simulink model "double_lwa4p_platform"  (R2020b)
settings: Solver=ode15s  StartTime=0.0  StopTime=T  MaxStep=0.01  RelTol=1e-3
values from neighbouring files (symbols this model uses):
  F_ee = [F_ee_A F_ee_B]    [sim_double_lwa4p_platform.m]
  friction = [fv1 fv2 fv3 fv4 fv5 fv6 fv1 fv2 fv3 fv4 fv5 fv6]    [sim_double_lwa4p_platform.m]
  g = [0 0 g0]'    [sim_double_lwa4p_platform.m]
  Kd = 5*eye(12)    [sim_double_lwa4p_platform.m]
  Kp = 2*eye(12)    [sim_double_lwa4p_platform.m]
  mass = [ml1 ml2 ml3 ml4 ml5 ml6 ml1 ml2 ml3 ml4 ml5 ml6]    [sim_double_lwa4p_platform.m]
  n_joints = 6    [sim_double_lwa4p_platform.m]
  q_ref = [pi/2 pi/4 pi/2 -pi/2 pi/2 -pi/8 pi/2 pi/4 pi/2 -pi/2 pi/2 -pi/8]    [sim_double_lwa4p_platform.m]
  qd_ref = zeros(1,12)    [sim_double_lwa4p_platform.m]
  qdd_ref = zeros(1,12)    [sim_double_lwa4p_platform.m]
  S = [S_A S_B]    [sim_double_lwa4p_platform.m]
  th1A_0 = deg2rad(0)    [sim_double_lwa4p_platform.m]
  th1B_0 = deg2rad(0)    [sim_double_lwa4p_platform.m]
  th2A_0 = deg2rad(0)    [sim_double_lwa4p_platform.m]
  th2B_0 = deg2rad(0)    [sim_double_lwa4p_platform.m]
  th3A_0 = deg2rad(0)    [sim_double_lwa4p_platform.m]
  th3B_0 = deg2rad(0)    [sim_double_lwa4p_platform.m]
  th4A_0 = deg2rad(0)    [sim_double_lwa4p_platform.m]
  th4B_0 = deg2rad(0)    [sim_double_lwa4p_platform.m]
  th5A_0 = deg2rad(0)    [sim_double_lwa4p_platform.m]
  th5B_0 = deg2rad(0)    [sim_double_lwa4p_platform.m]
  th6A_0 = deg2rad(0)    [sim_double_lwa4p_platform.m]
  th6B_0 = deg2rad(0)    [sim_double_lwa4p_platform.m]
undefined symbols (not defined in the file or in its folder): g0, Inertia, inertial_disp, ixx_1, ixx_2, ixx_3, ixx_4, ixx_5, ixx_6, ixx_platform, ixy_1, ixy_2, ixy_3, ixy_4, ixy_5, ixy_6, ixy_platform, ixz_1, ixz_2, ixz_3, ixz_4, ixz_5, ixz_6, ixz_platform, iyy_1, iyy_2, iyy_3, iyy_4, iyy_5, iyy_6, iyy_platform, iyz_1, iyz_2, iyz_3, iyz_4, iyz_5, iyz_6, iyz_platform, izz_1, izz_2, izz_3, izz_4, izz_5, izz_6, izz_platform, M_bi, m_platform, ml1, ml2, ml3, ml4, ml5, ml6, offA, offB, X, Y, Z
libraries: sm_lib x118, nesl_utility x49
(part 1 of 3)
settings Model: Creator=giank  LastModifiedBy=giank
settings ExplorerConfigSet: InternalSimMechanicsExplorerSettings="<ExplorerConfiguration><canonicalview>default</canonicalview><AnimationSetting><BasePlaybackSpeed>1.0</BasePlaybackSpeed><PlaybackSpeedFactor>1.0</PlaybackSpeedFactor></AnimationSetting><TilePanel><TileInfo><Tiles Columns=\"2\" Count=\"2\" Rows=\"1\"><Column Weight=\"0.4996\"/><Column Weight=\"0.5004\"/><Row Weight=\"1\"/><Tile Height=\"1\" Width=\"1\" X=\"0\" Y=\"0\"/><Tile Height=\"1\" Width=\"1\" X=\"1\" Y=\"0\"/></Tiles></TileInfo><SceneInfo><SceneViewer><BGColor><R>0.60000002384185791</R><G>0.60000002384185791</G><B>0.60000002384185791</B></BGColor><Camera><DoPerspective>off</DoPerspective><Position><X>-1.1818962679743017</X><Y>0.00783108174800895007</Y><Z>-0.680611997842788474</Z></Position><Center><X>1.20246335295615125e-05</X><Y>0.00783108174800895007</Y><Z>-0.680611997842788474</Z></Center><Up><X>0</X><Y>0</Y><Z>1</Z></Up><ViewLimDist>1</ViewLimDist><YLim>1.07089078664779658</YLim><XLim>0.814025905030074881</XLim></Camera></SceneViewer><SceneViewer><BGColor><R>0.60000002384185791</R><G>0.60000002384185791</G><B>0.60000002384185791</B></BGColor><Camera><DoPerspective>off</DoPerspective><Position><X>1.20351777254112946e-05</X><Y>-1.17407721146337618</Y><Z>-0.680611991448779152</Z></Position><Center><X>1.20351777254112946e-05</X><Y>0.00783108114445518755</Y><Z>-0.680611991448779152</Z></Center><Up><X>0</X><Y>-0</Y><Z>1</Z></Up><ViewLimDist>1</ViewLimDist><YLim>1.07089078664779658</YLim><XLim>0.816507691325898177</XLim></Camera></SceneViewer></SceneInfo></TilePanel><MechEditorPanel><Cameras/><GfxPanelCameraMap/><VideoCreator><PlaybackSpeedRatio>1.0</PlaybackSpeedRatio><FrameRate>30</FrameRate><VideoFormat>Motion JPEG AVI</VideoFormat><FrameSize>auto</FrameSize></VideoCreator></MechEditorPanel></ExplorerConfiguration>"

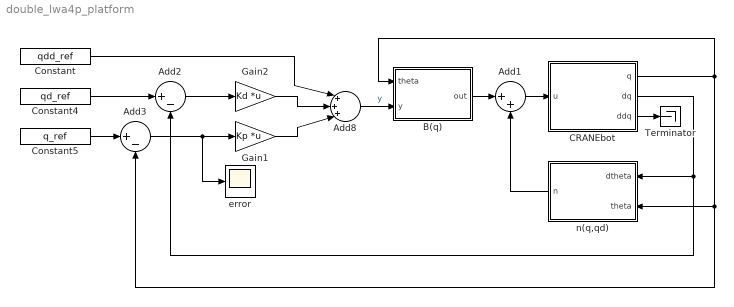
== system double_lwa4p_platform ==
  Add1 : Sum  Inputs=|++
  Add2 : Sum  Inputs=|+-
  Add3 : Sum  Inputs=|+-
  Add8 : Sum  Inputs=|+++|
  B(q) : MATLAB Function  TreatAsAtomicUnit=on
  CRANEbot : Subsystem
  Constant : Constant  Value=qdd_ref
  Constant4 : Constant  Value=qd_ref
  Constant5 : Constant  Value=q_ref
  Gain1 : Gain  Gain=Kp  Multiplication=Matrix(K*u)
  Gain2 : Gain  Gain=Kd  Multiplication=Matrix(K*u)
  Terminator : Terminator
  error : Scope
  n(q,qd) : MATLAB Function  TreatAsAtomicUnit=on
  wires:
  Gain1/1 -> Add8/3
  Add1/1 -> CRANEbot/1(u)
  CRANEbot/3(ddq) -> Terminator/1
  CRANEbot/2(dq) -> n(q,qd)/1(dtheta), Add2/2
  n(q,qd)/1(n) -> Add1/2
  Constant5/1 -> Add3/1
  B(q)/1(out) -> Add1/1
  Add8/1 -> B(q)/2(y)  "y"
  Constant4/1 -> Add2/1
  CRANEbot/1(q) -> n(q,qd)/2(theta), Add3/2, B(q)/1(theta)
  Add3/1 -> Gain1/1, error/1
  Constant/1 -> Add8/1
  Add2/1 -> Gain2/1
  Gain2/1 -> Add8/2

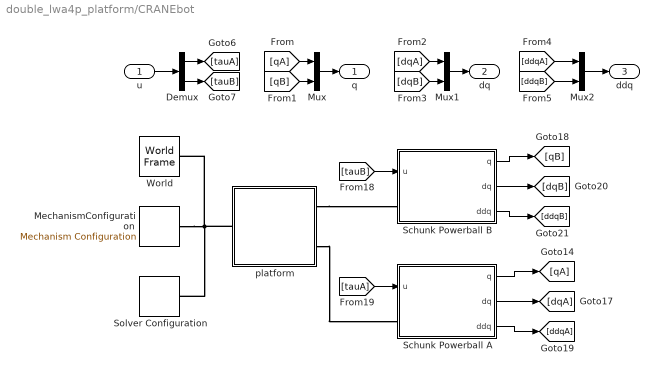
== system double_lwa4p_platform/CRANEbot ==
  u : Inport
  Demux : Demux  Outputs=[6 6 ]
  MechanismConfiguration : sm_lib/Utilities/Mechanism Configuration  UniformGravity=Constant  GravityVector=[0 0 -g0]  GravityVectorUnits=m/s^2  GravityUnits=m/s^2  LinearizationDelta=0.001  JointModeTransitionNonlinearIterations=2
  Mux : Mux  Inputs=[6 6]
  Mux1 : Mux  Inputs=[6 6]
  Mux2 : Mux  Inputs=[6 6]
  Schunk Powerball A : Subsystem  mask{th1_0=th1A_0, th2_0=th2A_0, th3_0=th3A_0, th4_0=th4A_0, th5_0=th5A_0, th6_0=th6A_0}
      mask prompts: th1_0 "th1_0 (rad)"; th2_0 "th2_0 (rad)"; th3_0 "th3_0 (rad)"; th4_0 "th4_0 (rad)"; th5_0 "th5_0 (rad)"; th6_0 "th6_0 (rad)"
  Schunk Powerball B : Subsystem  mask{th1_0=th1B_0, th2_0=th2B_0, th3_0=th3B_0, th4_0=th4B_0, th5_0=th5B_0, th6_0=th6B_0}
      mask prompts: th1_0 "th1_0 (rad)"; th2_0 "th2_0 (rad)"; th3_0 "th3_0 (rad)"; th4_0 "th4_0 (rad)"; th5_0 "th5_0 (rad)"; th6_0 "th6_0 (rad)"
  Solver Configuration : nesl_utility/Solver Configuration  PhysicalDomain=network_engine_domain  SubClassName=solver  LeftPortType=input  RightPortType=generic  Tones=[]  Harmonics=[]  SimulateNoise=off  Profile=off  UseLocalSampling=off  EnableSwitchedLinearOptims=on  FrequencyDomain=off  UseCCode=off  RelTol=0.001  AbsTol=1e-06  MinStep=1e-09  ToWorkspace=off  RevertToSquareIcSolve=off  NumHomotopyIterations=100  PhasorMode=off  PhasorModeNumHarmonics=1  DoDC=off  ResidualTolerance=1e-09  UseLocalSolver=off  LocalSolverChoice=NE_BACKWARD_EULER_ADVANCER  LocalSolverSampleTime=0.001  DoFixedCost=off  MaxNonlinIter=3  MaxModeIter=2  ComputeImpulses=off  ImpulseIterations=2  LinearAlgebra=auto  EquationFormulation=NE_TIME_EF  DelaysMemoryBudget=1024  AutomaticFiltering=on  FilteringTimeConstant=0.001  PartitionStorageMethod=AS_NEEDED  PartitionMemoryBudget=1024  PartitionMethod=ROBUST
  World : sm_lib/Frames and Transforms/World Frame
  platform : Subsystem
  q : Outport
  dq : Outport  Port=2
  ddq : Outport  Port=3
  wires:
  Mux/1 -> q/1
  [qA] -> Mux/1
  Mux1/1 -> dq/1
  u/1 -> Demux/1
  [qB] -> Mux/2
  Demux/1 -> [tauA]
  [dqB] -> Mux1/2
  Demux/2 -> [tauB]
  Mux2/1 -> ddq/1
  [ddqA] -> Mux2/1
  [dqA] -> Mux1/1
  [ddqB] -> Mux2/2
  Schunk Powerball B/2(dq) -> [dqB]
  Schunk Powerball A/1(q) -> [qA]
  Schunk Powerball B/3(ddq) -> [ddqB]
  Schunk Powerball A/2(dq) -> [dqA]
  [tauB] -> Schunk Powerball B/1(u)
  Schunk Powerball A/3(ddq) -> [ddqA]
  [tauA] -> Schunk Powerball A/1(u)
  Schunk Powerball B/1(q) -> [qB]
  connections:
  Solver Configuration/RConn1 -- platform/LConn1 -- World/RConn1 -- MechanismConfiguration/RConn1
  platform/RConn1 -- Schunk Powerball B/LConn1
  platform/RConn2 -- Schunk Powerball A/LConn1

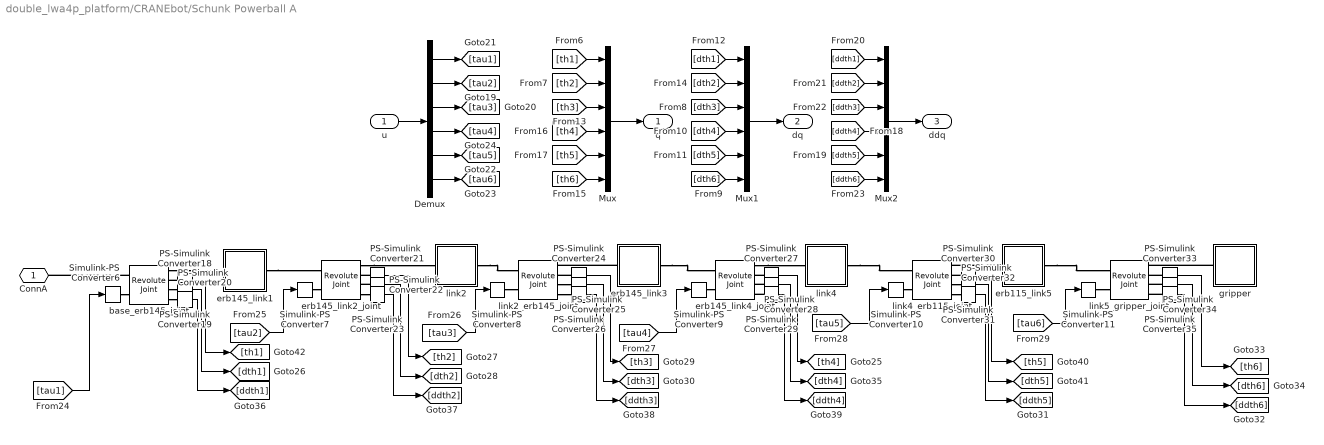
== system double_lwa4p_platform/CRANEbot/Schunk Powerball A ==
  u : Inport
  Demux : Demux  Outputs=6
  Mux : Mux  Inputs=6
  Mux1 : Mux  Inputs=6
  Mux2 : Mux  Inputs=6
  PS-Simulink Converter{18..35} (18 alike) : nesl_utility/PS-Simulink Converter  PhysicalDomain=network_engine_domain  SubClassName=ps_output  LeftPortType=input  RightPortType=output  PseudoPeriodic=off  Frequencies=[]  Unit=inherit  AffineConversion=off
  Simulink-PS Converter{6..11} (6 alike) : nesl_utility/Simulink-PS Converter  PhysicalDomain=network_engine_domain  SubClassName=ps_input  LeftPortType=input  RightPortType=output  PseudoPeriodic=off  Frequencies=[]  NoiseDistribution=none  NoiseParameters=[]  Unit=1  AffineConversion=off  FilteringAndDerivatives=provide  SimscapeFilterOrder=1  InputFilterTimeConstant=0.001  UdotUserProvided=0
  base_erb145_joint : sm_lib/Joints/Revolute Joint  JointMode=Normal  SenseConstraintForce=off  SenseConstraintForceX=off  SenseConstraintForceY=off  SenseConstraintForceZ=off  SenseConstraintTorque=off  SenseConstraintTorqueX=off  SenseConstraintTorqueY=off  SenseConstraintTorqueZ=off  SenseTotalForce=off  SenseTotalForceX=off  SenseTotalForceY=off  SenseTotalForceZ=off  SenseTotalTorque=off  SenseTotalTorqueX=off  SenseTotalTorqueY=off  SenseTotalTorqueZ=off  CompositeWrenchDir=FollowerOnBase  CompositeWrenchFrame=BaseFrame  EquilibriumPosition=0  EquilibriumPositionUnits=deg  SpringStiffness=0  SpringStiffnessUnits=N*m/deg  DampingCoefficient=fv1  DampingCoefficientUnits=N*m/(rad/s)  TorqueActuationMode=InputTorque  MotionActuationMode=ComputedMotion  SensePosition=on  SenseVelocity=on  SenseAcceleration=on  SenseTorqueForce=off  SenseLowerLimitTorqueForce=off  SenseUpperLimitTorqueForce=off  LowerLimitSpecify=on  LowerLimitBound=J1_lower_limit  LowerLimitBoundUnits=deg  LowerLimitStiffness=1e4  LowerLimitStiffnessUnits=N*m/deg  LowerLimitDamping=10  LowerLimitDampingUnits=N*m/(deg/s)  LowerLimitTransitionRegionWidth=0.1  LowerLimitTransitionRegionWidthUnits=deg  UpperLimitSpecify=on  UpperLimitBound=J1_upper_limit  UpperLimitBoundUnits=deg  UpperLimitStiffness=1e4  UpperLimitStiffnessUnits=N*m/deg  UpperLimitDamping=10  UpperLimitDampingUnits=N*m/(deg/s)  UpperLimitTransitionRegionWidth=0.1  UpperLimitTransitionRegionWidthUnits=deg  PositionTargetSpecify=on  PositionTargetPriority=High  PositionTargetValue=th1_0  PositionTargetValueUnits=rad  VelocityTargetSpecify=off  VelocityTargetPriority=High  VelocityTargetValue=0  VelocityTargetValueUnits=deg/s
  erb115_link5 : Subsystem
  erb145_link1 : Subsystem
  erb145_link2_joint : sm_lib/Joints/Revolute Joint  JointMode=Normal  SenseConstraintForce=off  SenseConstraintForceX=off  SenseConstraintForceY=off  SenseConstraintForceZ=off  SenseConstraintTorque=off  SenseConstraintTorqueX=off  SenseConstraintTorqueY=off  SenseConstraintTorqueZ=off  SenseTotalForce=off  SenseTotalForceX=off  SenseTotalForceY=off  SenseTotalForceZ=off  SenseTotalTorque=off  SenseTotalTorqueX=off  SenseTotalTorqueY=off  SenseTotalTorqueZ=off  CompositeWrenchDir=FollowerOnBase  CompositeWrenchFrame=BaseFrame  EquilibriumPosition=0  EquilibriumPositionUnits=deg  SpringStiffness=0  SpringStiffnessUnits=N*m/deg  DampingCoefficient=fv2  DampingCoefficientUnits=N*m/(rad/s)  TorqueActuationMode=InputTorque  MotionActuationMode=ComputedMotion  SensePosition=on  SenseVelocity=on  SenseAcceleration=on  SenseTorqueForce=off  SenseLowerLimitTorqueForce=off  SenseUpperLimitTorqueForce=off  LowerLimitSpecify=on  LowerLimitBound=J2_lower_limit  LowerLimitBoundUnits=deg  LowerLimitStiffness=1e4  LowerLimitStiffnessUnits=N*m/deg  LowerLimitDamping=10  LowerLimitDampingUnits=N*m/(deg/s)  LowerLimitTransitionRegionWidth=0.1  LowerLimitTransitionRegionWidthUnits=deg  UpperLimitSpecify=on  UpperLimitBound=J2_upper_limit  UpperLimitBoundUnits=deg  UpperLimitStiffness=1e4  UpperLimitStiffnessUnits=N*m/deg  UpperLimitDamping=10  UpperLimitDampingUnits=N*m/(deg/s)  UpperLimitTransitionRegionWidth=0.1  UpperLimitTransitionRegionWidthUnits=deg  PositionTargetSpecify=on  PositionTargetPriority=High  PositionTargetValue=th2_0  PositionTargetValueUnits=deg  VelocityTargetSpecify=off  VelocityTargetPriority=High  VelocityTargetValue=0  VelocityTargetValueUnits=deg/s
  erb145_link3 : Subsystem
  erb145_link4_joint : sm_lib/Joints/Revolute Joint  JointMode=Normal  SenseConstraintForce=off  SenseConstraintForceX=off  SenseConstraintForceY=off  SenseConstraintForceZ=off  SenseConstraintTorque=off  SenseConstraintTorqueX=off  SenseConstraintTorqueY=off  SenseConstraintTorqueZ=off  SenseTotalForce=off  SenseTotalForceX=off  SenseTotalForceY=off  SenseTotalForceZ=off  SenseTotalTorque=off  SenseTotalTorqueX=off  SenseTotalTorqueY=off  SenseTotalTorqueZ=off  CompositeWrenchDir=FollowerOnBase  CompositeWrenchFrame=BaseFrame  EquilibriumPosition=0  EquilibriumPositionUnits=deg  SpringStiffness=0  SpringStiffnessUnits=N*m/deg  DampingCoefficient=fv4  DampingCoefficientUnits=N*m/(rad/s)  TorqueActuationMode=InputTorque  MotionActuationMode=ComputedMotion  SensePosition=on  SenseVelocity=on  SenseAcceleration=on  SenseTorqueForce=off  SenseLowerLimitTorqueForce=off  SenseUpperLimitTorqueForce=off  LowerLimitSpecify=on  LowerLimitBound=J4_lower_limit  LowerLimitBoundUnits=deg  LowerLimitStiffness=1e4  LowerLimitStiffnessUnits=N*m/deg  LowerLimitDamping=10  LowerLimitDampingUnits=N*m/(deg/s)  LowerLimitTransitionRegionWidth=0.1  LowerLimitTransitionRegionWidthUnits=deg  UpperLimitSpecify=on  UpperLimitBound=J4_upper_limit  UpperLimitBoundUnits=deg  UpperLimitStiffness=1e4  UpperLimitStiffnessUnits=N*m/deg  UpperLimitDamping=10  UpperLimitDampingUnits=N*m/(deg/s)  UpperLimitTransitionRegionWidth=0.1  UpperLimitTransitionRegionWidthUnits=deg  PositionTargetSpecify=on  PositionTargetPriority=High  PositionTargetValue=th4_0  PositionTargetValueUnits=deg  VelocityTargetSpecify=off  VelocityTargetPriority=High  VelocityTargetValue=0  VelocityTargetValueUnits=deg/s
  gripper : Subsystem
  link2 : Subsystem
  link2_erb145_joint : sm_lib/Joints/Revolute Joint  JointMode=Normal  SenseConstraintForce=off  SenseConstraintForceX=off  SenseConstraintForceY=off  SenseConstraintForceZ=off  SenseConstraintTorque=off  SenseConstraintTorqueX=off  SenseConstraintTorqueY=off  SenseConstraintTorqueZ=off  SenseTotalForce=off  SenseTotalForceX=off  SenseTotalForceY=off  SenseTotalForceZ=off  SenseTotalTorque=off  SenseTotalTorqueX=off  SenseTotalTorqueY=off  SenseTotalTorqueZ=off  CompositeWrenchDir=FollowerOnBase  CompositeWrenchFrame=BaseFrame  EquilibriumPosition=0  EquilibriumPositionUnits=deg  SpringStiffness=0  SpringStiffnessUnits=N*m/deg  DampingCoefficient=fv3  DampingCoefficientUnits=N*m/(rad/s)  TorqueActuationMode=InputTorque  MotionActuationMode=ComputedMotion  SensePosition=on  SenseVelocity=on  SenseAcceleration=on  SenseTorqueForce=off  SenseLowerLimitTorqueForce=off  SenseUpperLimitTorqueForce=off  LowerLimitSpecify=on  LowerLimitBound=J3_lower_limit  LowerLimitBoundUnits=deg  LowerLimitStiffness=1e4  LowerLimitStiffnessUnits=N*m/deg  LowerLimitDamping=10  LowerLimitDampingUnits=N*m/(deg/s)  LowerLimitTransitionRegionWidth=0.1  LowerLimitTransitionRegionWidthUnits=deg  UpperLimitSpecify=on  UpperLimitBound=J3_upper_limit  UpperLimitBoundUnits=deg  UpperLimitStiffness=1e4  UpperLimitStiffnessUnits=N*m/deg  UpperLimitDamping=10  UpperLimitDampingUnits=N*m/(deg/s)  UpperLimitTransitionRegionWidth=0.1  UpperLimitTransitionRegionWidthUnits=deg  PositionTargetSpecify=on  PositionTargetPriority=High  PositionTargetValue=th3_0  PositionTargetValueUnits=deg  VelocityTargetSpecify=off  VelocityTargetPriority=High  VelocityTargetValue=0  VelocityTargetValueUnits=deg/s
  link4 : Subsystem
  link4_erb115_joint : sm_lib/Joints/Revolute Joint  JointMode=Normal  SenseConstraintForce=off  SenseConstraintForceX=off  SenseConstraintForceY=off  SenseConstraintForceZ=off  SenseConstraintTorque=off  SenseConstraintTorqueX=off  SenseConstraintTorqueY=off  SenseConstraintTorqueZ=off  SenseTotalForce=off  SenseTotalForceX=off  SenseTotalForceY=off  SenseTotalForceZ=off  SenseTotalTorque=off  SenseTotalTorqueX=off  SenseTotalTorqueY=off  SenseTotalTorqueZ=off  CompositeWrenchDir=FollowerOnBase  CompositeWrenchFrame=BaseFrame  EquilibriumPosition=0  EquilibriumPositionUnits=deg  SpringStiffness=0  SpringStiffnessUnits=N*m/deg  DampingCoefficient=fv5  DampingCoefficientUnits=N*m/(rad/s)  TorqueActuationMode=InputTorque  MotionActuationMode=ComputedMotion  SensePosition=on  SenseVelocity=on  SenseAcceleration=on  SenseTorqueForce=off  SenseLowerLimitTorqueForce=off  SenseUpperLimitTorqueForce=off  LowerLimitSpecify=on  LowerLimitBound=J5_lower_limit  LowerLimitBoundUnits=deg  LowerLimitStiffness=1e4  LowerLimitStiffnessUnits=N*m/deg  LowerLimitDamping=10  LowerLimitDampingUnits=N*m/(deg/s)  LowerLimitTransitionRegionWidth=0.1  LowerLimitTransitionRegionWidthUnits=deg  UpperLimitSpecify=on  UpperLimitBound=J5_upper_limit  UpperLimitBoundUnits=deg  UpperLimitStiffness=1e4  UpperLimitStiffnessUnits=N*m/deg  UpperLimitDamping=10  UpperLimitDampingUnits=N*m/(deg/s)  UpperLimitTransitionRegionWidth=0.1  UpperLimitTransitionRegionWidthUnits=deg  PositionTargetSpecify=on  PositionTargetPriority=High  PositionTargetValue=th5_0  PositionTargetValueUnits=deg  VelocityTargetSpecify=off  VelocityTargetPriority=High  VelocityTargetValue=0  VelocityTargetValueUnits=deg/s
  link5_gripper_joint : sm_lib/Joints/Revolute Joint  JointMode=Normal  SenseConstraintForce=off  SenseConstraintForceX=off  SenseConstraintForceY=off  SenseConstraintForceZ=off  SenseConstraintTorque=off  SenseConstraintTorqueX=off  SenseConstraintTorqueY=off  SenseConstraintTorqueZ=off  SenseTotalForce=off  SenseTotalForceX=off  SenseTotalForceY=off  SenseTotalForceZ=off  SenseTotalTorque=off  SenseTotalTorqueX=off  SenseTotalTorqueY=off  SenseTotalTorqueZ=off  CompositeWrenchDir=FollowerOnBase  CompositeWrenchFrame=BaseFrame  EquilibriumPosition=0  EquilibriumPositionUnits=deg  SpringStiffness=0  SpringStiffnessUnits=N*m/deg  DampingCoefficient=fv6  DampingCoefficientUnits=N*m/(rad/s)  TorqueActuationMode=InputTorque  MotionActuationMode=ComputedMotion  SensePosition=on  SenseVelocity=on  SenseAcceleration=on  SenseTorqueForce=off  SenseLowerLimitTorqueForce=off  SenseUpperLimitTorqueForce=off  LowerLimitSpecify=on  LowerLimitBound=J6_lower_limit  LowerLimitBoundUnits=deg  LowerLimitStiffness=1e4  LowerLimitStiffnessUnits=N*m/deg  LowerLimitDamping=10  LowerLimitDampingUnits=N*m/(deg/s)  LowerLimitTransitionRegionWidth=0.1  LowerLimitTransitionRegionWidthUnits=deg  UpperLimitSpecify=on  UpperLimitBound=J6_upper_limit  UpperLimitBoundUnits=deg  UpperLimitStiffness=1e4  UpperLimitStiffnessUnits=N*m/deg  UpperLimitDamping=10  UpperLimitDampingUnits=N*m/(deg/s)  UpperLimitTransitionRegionWidth=0.1  UpperLimitTransitionRegionWidthUnits=deg  PositionTargetSpecify=on  PositionTargetPriority=High  PositionTargetValue=th6_0  PositionTargetValueUnits=deg  VelocityTargetSpecify=off  VelocityTargetPriority=High  VelocityTargetValue=0  VelocityTargetValueUnits=deg/s
  ConnA : PMIOPort  Side=Left
  q : Outport
  dq : Outport  Port=2
  ddq : Outport  Port=3
  wires:
  [tau6] -> Simulink-PS Converter11/1
  PS-Simulink Converter22/1 -> [dth2]
  Demux/2 -> [tau2]
  [ddth6] -> Mux2/6
  PS-Simulink Converter28/1 -> [dth4]
  [dth2] -> Mux1/2
  Demux/5 -> [tau5]
  [tau4] -> Simulink-PS Converter9/1
  PS-Simulink Converter30/1 -> [th5]
  PS-Simulink Converter19/1 -> [dth1]
  [th3] -> Mux/3
  PS-Simulink Converter34/1 -> [dth6]
  PS-Simulink Converter26/1 -> [ddth3]
  PS-Simulink Converter24/1 -> [th3]
  PS-Simulink Converter25/1 -> [dth3]
  PS-Simulink Converter31/1 -> [dth5]
  PS-Simulink Converter27/1 -> [th4]
  [dth3] -> Mux1/3
  [th1] -> Mux/1
  PS-Simulink Converter33/1 -> [th6]
  u/1 -> Demux/1
  [th2] -> Mux/2
  [ddth3] -> Mux2/3
  Demux/6 -> [tau6]
  PS-Simulink Converter20/1 -> [ddth1]
  Mux/1 -> q/1
  PS-Simulink Converter18/1 -> [th1]
  [ddth4] -> Mux2/4
  PS-Simulink Converter29/1 -> [ddth4]
  [ddth2] -> Mux2/2
  [dth1] -> Mux1/1
  [dth5] -> Mux1/5
  Demux/4 -> [tau4]
  [dth4] -> Mux1/4
  [dth6] -> Mux1/6
  PS-Simulink Converter23/1 -> [ddth2]
  [th5] -> Mux/5
  [ddth5] -> Mux2/5
  [th4] -> Mux/4
  Mux2/1 -> ddq/1
  PS-Simulink Converter21/1 -> [th2]
  Mux1/1 -> dq/1
  [ddth1] -> Mux2/1
  Demux/3 -> [tau3]
  PS-Simulink Converter32/1 -> [ddth5]
  [tau2] -> Simulink-PS Converter7/1
  [tau3] -> Simulink-PS Converter8/1
  Demux/1 -> [tau1]
  [tau5] -> Simulink-PS Converter10/1
  [tau1] -> Simulink-PS Converter6/1
  PS-Simulink Converter35/1 -> [ddth6]
  [th6] -> Mux/6
  connections:
  erb145_link1/RConn1 -- erb145_link2_joint/LConn1
  erb115_link5/RConn1 -- link5_gripper_joint/LConn1
  Simulink-PS Converter9/RConn1 -- erb145_link4_joint/LConn2
  base_erb145_joint/LConn1 -- ConnA/RConn1
  base_erb145_joint/RConn1 -- erb145_link1/LConn1
  Simulink-PS Converter7/RConn1 -- erb145_link2_joint/LConn2
  PS-Simulink Converter18/LConn1 -- base_erb145_joint/RConn2
  erb145_link3/LConn1 -- link2_erb145_joint/RConn1
  Simulink-PS Converter6/RConn1 -- base_erb145_joint/LConn2
  link2_erb145_joint/RConn3 -- PS-Simulink Converter25/LConn1
  link2_erb145_joint/RConn4 -- PS-Simulink Converter26/LConn1
  PS-Simulink Converter21/LConn1 -- erb145_link2_joint/RConn2
  PS-Simulink Converter33/LConn1 -- link5_gripper_joint/RConn2
  PS-Simulink Converter22/LConn1 -- erb145_link2_joint/RConn3
  link2/RConn1 -- link2_erb145_joint/LConn1
  Simulink-PS Converter8/RConn1 -- link2_erb145_joint/LConn2
  erb115_link5/LConn1 -- link4_erb115_joint/RConn1
  erb145_link2_joint/RConn1 -- link2/LConn1
  PS-Simulink Converter28/LConn1 -- erb145_link4_joint/RConn3
  PS-Simulink Converter35/LConn1 -- link5_gripper_joint/RConn4
  PS-Simulink Converter29/LConn1 -- erb145_link4_joint/RConn4
  Simulink-PS Converter10/RConn1 -- link4_erb115_joint/LConn2
  PS-Simulink Converter30/LConn1 -- link4_erb115_joint/RConn2
  base_erb145_joint/RConn3 -- PS-Simulink Converter19/LConn1
  erb145_link2_joint/RConn4 -- PS-Simulink Converter23/LConn1
  link4/RConn1 -- link4_erb115_joint/LConn1
  link4_erb115_joint/RConn4 -- PS-Simulink Converter32/LConn1
  erb145_link4_joint/RConn1 -- link4/LConn1
  PS-Simulink Converter24/LConn1 -- link2_erb145_joint/RConn2
  Simulink-PS Converter11/RConn1 -- link5_gripper_joint/LConn2
  PS-Simulink Converter34/LConn1 -- link5_gripper_joint/RConn3
  erb145_link3/RConn1 -- erb145_link4_joint/LConn1
  PS-Simulink Converter27/LConn1 -- erb145_link4_joint/RConn2
  link4_erb115_joint/RConn3 -- PS-Simulink Converter31/LConn1
  gripper/LConn1 -- link5_gripper_joint/RConn1
  base_erb145_joint/RConn4 -- PS-Simulink Converter20/LConn1

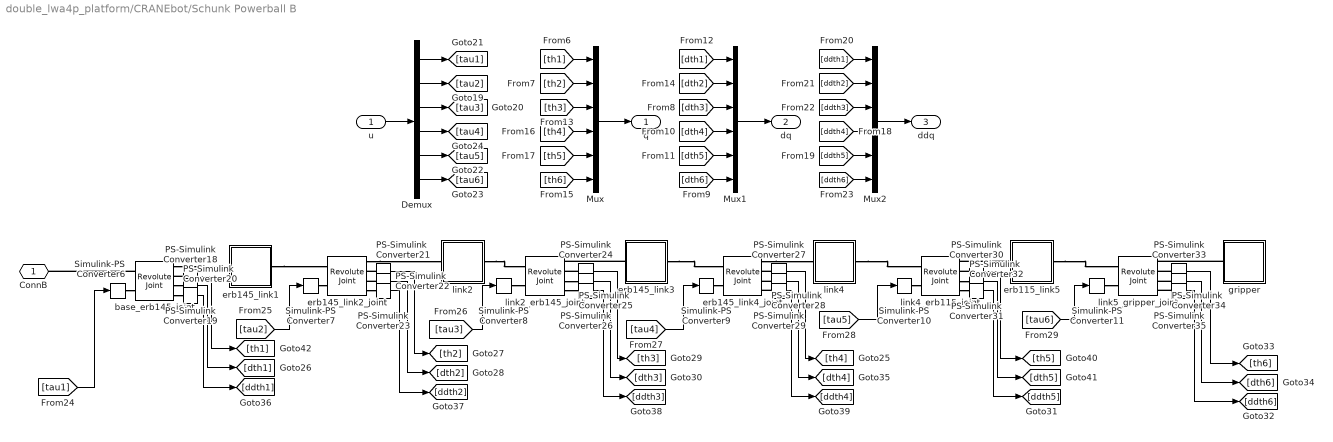
== system double_lwa4p_platform/CRANEbot/Schunk Powerball B ==
  u : Inport
  Demux : Demux  Outputs=6
  Mux : Mux  Inputs=6
  Mux1 : Mux  Inputs=6
  Mux2 : Mux  Inputs=6
  PS-Simulink Converter{18..35} (18 alike) : nesl_utility/PS-Simulink Converter  PhysicalDomain=network_engine_domain  SubClassName=ps_output  LeftPortType=input  RightPortType=output  PseudoPeriodic=off  Frequencies=[]  Unit=inherit  AffineConversion=off
  Simulink-PS Converter{6..11} (6 alike) : nesl_utility/Simulink-PS Converter  PhysicalDomain=network_engine_domain  SubClassName=ps_input  LeftPortType=input  RightPortType=output  PseudoPeriodic=off  Frequencies=[]  NoiseDistribution=none  NoiseParameters=[]  Unit=1  AffineConversion=off  FilteringAndDerivatives=provide  SimscapeFilterOrder=1  InputFilterTimeConstant=0.001  UdotUserProvided=0
  base_erb145_joint : sm_lib/Joints/Revolute Joint  JointMode=Normal  SenseConstraintForce=off  SenseConstraintForceX=off  SenseConstraintForceY=off  SenseConstraintForceZ=off  SenseConstraintTorque=off  SenseConstraintTorqueX=off  SenseConstraintTorqueY=off  SenseConstraintTorqueZ=off  SenseTotalForce=off  SenseTotalForceX=off  SenseTotalForceY=off  SenseTotalForceZ=off  SenseTotalTorque=off  SenseTotalTorqueX=off  SenseTotalTorqueY=off  SenseTotalTorqueZ=off  CompositeWrenchDir=FollowerOnBase  CompositeWrenchFrame=BaseFrame  EquilibriumPosition=0  EquilibriumPositionUnits=deg  SpringStiffness=0  SpringStiffnessUnits=N*m/deg  DampingCoefficient=fv1  DampingCoefficientUnits=N*m/(rad/s)  TorqueActuationMode=InputTorque  MotionActuationMode=ComputedMotion  SensePosition=on  SenseVelocity=on  SenseAcceleration=on  SenseTorqueForce=off  SenseLowerLimitTorqueForce=off  SenseUpperLimitTorqueForce=off  LowerLimitSpecify=on  LowerLimitBound=J1_lower_limit  LowerLimitBoundUnits=deg  LowerLimitStiffness=1e4  LowerLimitStiffnessUnits=N*m/deg  LowerLimitDamping=10  LowerLimitDampingUnits=N*m/(deg/s)  LowerLimitTransitionRegionWidth=0.1  LowerLimitTransitionRegionWidthUnits=deg  UpperLimitSpecify=on  UpperLimitBound=J1_upper_limit  UpperLimitBoundUnits=deg  UpperLimitStiffness=1e4  UpperLimitStiffnessUnits=N*m/deg  UpperLimitDamping=10  UpperLimitDampingUnits=N*m/(deg/s)  UpperLimitTransitionRegionWidth=0.1  UpperLimitTransitionRegionWidthUnits=deg  PositionTargetSpecify=on  PositionTargetPriority=High  PositionTargetValue=th1_0  PositionTargetValueUnits=rad  VelocityTargetSpecify=off  VelocityTargetPriority=High  VelocityTargetValue=0  VelocityTargetValueUnits=deg/s
  erb115_link5 : Subsystem
  erb145_link1 : Subsystem
  erb145_link2_joint : sm_lib/Joints/Revolute Joint  JointMode=Normal  SenseConstraintForce=off  SenseConstraintForceX=off  SenseConstraintForceY=off  SenseConstraintForceZ=off  SenseConstraintTorque=off  SenseConstraintTorqueX=off  SenseConstraintTorqueY=off  SenseConstraintTorqueZ=off  SenseTotalForce=off  SenseTotalForceX=off  SenseTotalForceY=off  SenseTotalForceZ=off  SenseTotalTorque=off  SenseTotalTorqueX=off  SenseTotalTorqueY=off  SenseTotalTorqueZ=off  CompositeWrenchDir=FollowerOnBase  CompositeWrenchFrame=BaseFrame  EquilibriumPosition=0  EquilibriumPositionUnits=deg  SpringStiffness=0  SpringStiffnessUnits=N*m/deg  DampingCoefficient=fv2  DampingCoefficientUnits=N*m/(rad/s)  TorqueActuationMode=InputTorque  MotionActuationMode=ComputedMotion  SensePosition=on  SenseVelocity=on  SenseAcceleration=on  SenseTorqueForce=off  SenseLowerLimitTorqueForce=off  SenseUpperLimitTorqueForce=off  LowerLimitSpecify=on  LowerLimitBound=J2_lower_limit  LowerLimitBoundUnits=deg  LowerLimitStiffness=1e4  LowerLimitStiffnessUnits=N*m/deg  LowerLimitDamping=10  LowerLimitDampingUnits=N*m/(deg/s)  LowerLimitTransitionRegionWidth=0.1  LowerLimitTransitionRegionWidthUnits=deg  UpperLimitSpecify=on  UpperLimitBound=J2_upper_limit  UpperLimitBoundUnits=deg  UpperLimitStiffness=1e4  UpperLimitStiffnessUnits=N*m/deg  UpperLimitDamping=10  UpperLimitDampingUnits=N*m/(deg/s)  UpperLimitTransitionRegionWidth=0.1  UpperLimitTransitionRegionWidthUnits=deg  PositionTargetSpecify=on  PositionTargetPriority=High  PositionTargetValue=th2_0  PositionTargetValueUnits=deg  VelocityTargetSpecify=off  VelocityTargetPriority=High  VelocityTargetValue=0  VelocityTargetValueUnits=deg/s
  erb145_link3 : Subsystem
  erb145_link4_joint : sm_lib/Joints/Revolute Joint  JointMode=Normal  SenseConstraintForce=off  SenseConstraintForceX=off  SenseConstraintForceY=off  SenseConstraintForceZ=off  SenseConstraintTorque=off  SenseConstraintTorqueX=off  SenseConstraintTorqueY=off  SenseConstraintTorqueZ=off  SenseTotalForce=off  SenseTotalForceX=off  SenseTotalForceY=off  SenseTotalForceZ=off  SenseTotalTorque=off  SenseTotalTorqueX=off  SenseTotalTorqueY=off  SenseTotalTorqueZ=off  CompositeWrenchDir=FollowerOnBase  CompositeWrenchFrame=BaseFrame  EquilibriumPosition=0  EquilibriumPositionUnits=deg  SpringStiffness=0  SpringStiffnessUnits=N*m/deg  DampingCoefficient=fv4  DampingCoefficientUnits=N*m/(rad/s)  TorqueActuationMode=InputTorque  MotionActuationMode=ComputedMotion  SensePosition=on  SenseVelocity=on  SenseAcceleration=on  SenseTorqueForce=off  SenseLowerLimitTorqueForce=off  SenseUpperLimitTorqueForce=off  LowerLimitSpecify=on  LowerLimitBound=J4_lower_limit  LowerLimitBoundUnits=deg  LowerLimitStiffness=1e4  LowerLimitStiffnessUnits=N*m/deg  LowerLimitDamping=10  LowerLimitDampingUnits=N*m/(deg/s)  LowerLimitTransitionRegionWidth=0.1  LowerLimitTransitionRegionWidthUnits=deg  UpperLimitSpecify=on  UpperLimitBound=J4_upper_limit  UpperLimitBoundUnits=deg  UpperLimitStiffness=1e4  UpperLimitStiffnessUnits=N*m/deg  UpperLimitDamping=10  UpperLimitDampingUnits=N*m/(deg/s)  UpperLimitTransitionRegionWidth=0.1  UpperLimitTransitionRegionWidthUnits=deg  PositionTargetSpecify=on  PositionTargetPriority=High  PositionTargetValue=th4_0  PositionTargetValueUnits=deg  VelocityTargetSpecify=off  VelocityTargetPriority=High  VelocityTargetValue=0  VelocityTargetValueUnits=deg/s
  gripper : Subsystem
  link2 : Subsystem
  link2_erb145_joint : sm_lib/Joints/Revolute Joint  JointMode=Normal  SenseConstraintForce=off  SenseConstraintForceX=off  SenseConstraintForceY=off  SenseConstraintForceZ=off  SenseConstraintTorque=off  SenseConstraintTorqueX=off  SenseConstraintTorqueY=off  SenseConstraintTorqueZ=off  SenseTotalForce=off  SenseTotalForceX=off  SenseTotalForceY=off  SenseTotalForceZ=off  SenseTotalTorque=off  SenseTotalTorqueX=off  SenseTotalTorqueY=off  SenseTotalTorqueZ=off  CompositeWrenchDir=FollowerOnBase  CompositeWrenchFrame=BaseFrame  EquilibriumPosition=0  EquilibriumPositionUnits=deg  SpringStiffness=0  SpringStiffnessUnits=N*m/deg  DampingCoefficient=fv3  DampingCoefficientUnits=N*m/(rad/s)  TorqueActuationMode=InputTorque  MotionActuationMode=ComputedMotion  SensePosition=on  SenseVelocity=on  SenseAcceleration=on  SenseTorqueForce=off  SenseLowerLimitTorqueForce=off  SenseUpperLimitTorqueForce=off  LowerLimitSpecify=on  LowerLimitBound=J3_lower_limit  LowerLimitBoundUnits=deg  LowerLimitStiffness=1e4  LowerLimitStiffnessUnits=N*m/deg  LowerLimitDamping=10  LowerLimitDampingUnits=N*m/(deg/s)  LowerLimitTransitionRegionWidth=0.1  LowerLimitTransitionRegionWidthUnits=deg  UpperLimitSpecify=on  UpperLimitBound=J3_upper_limit  UpperLimitBoundUnits=deg  UpperLimitStiffness=1e4  UpperLimitStiffnessUnits=N*m/deg  UpperLimitDamping=10  UpperLimitDampingUnits=N*m/(deg/s)  UpperLimitTransitionRegionWidth=0.1  UpperLimitTransitionRegionWidthUnits=deg  PositionTargetSpecify=on  PositionTargetPriority=High  PositionTargetValue=th3_0  PositionTargetValueUnits=deg  VelocityTargetSpecify=off  VelocityTargetPriority=High  VelocityTargetValue=0  VelocityTargetValueUnits=deg/s
  link4 : Subsystem
  link4_erb115_joint : sm_lib/Joints/Revolute Joint  JointMode=Normal  SenseConstraintForce=off  SenseConstraintForceX=off  SenseConstraintForceY=off  SenseConstraintForceZ=off  SenseConstraintTorque=off  SenseConstraintTorqueX=off  SenseConstraintTorqueY=off  SenseConstraintTorqueZ=off  SenseTotalForce=off  SenseTotalForceX=off  SenseTotalForceY=off  SenseTotalForceZ=off  SenseTotalTorque=off  SenseTotalTorqueX=off  SenseTotalTorqueY=off  SenseTotalTorqueZ=off  CompositeWrenchDir=FollowerOnBase  CompositeWrenchFrame=BaseFrame  EquilibriumPosition=0  EquilibriumPositionUnits=deg  SpringStiffness=0  SpringStiffnessUnits=N*m/deg  DampingCoefficient=fv5  DampingCoefficientUnits=N*m/(rad/s)  TorqueActuationMode=InputTorque  MotionActuationMode=ComputedMotion  SensePosition=on  SenseVelocity=on  SenseAcceleration=on  SenseTorqueForce=off  SenseLowerLimitTorqueForce=off  SenseUpperLimitTorqueForce=off  LowerLimitSpecify=on  LowerLimitBound=J5_lower_limit  LowerLimitBoundUnits=deg  LowerLimitStiffness=1e4  LowerLimitStiffnessUnits=N*m/deg  LowerLimitDamping=10  LowerLimitDampingUnits=N*m/(deg/s)  LowerLimitTransitionRegionWidth=0.1  LowerLimitTransitionRegionWidthUnits=deg  UpperLimitSpecify=on  UpperLimitBound=J5_upper_limit  UpperLimitBoundUnits=deg  UpperLimitStiffness=1e4  UpperLimitStiffnessUnits=N*m/deg  UpperLimitDamping=10  UpperLimitDampingUnits=N*m/(deg/s)  UpperLimitTransitionRegionWidth=0.1  UpperLimitTransitionRegionWidthUnits=deg  PositionTargetSpecify=on  PositionTargetPriority=High  PositionTargetValue=th5_0  PositionTargetValueUnits=deg  VelocityTargetSpecify=off  VelocityTargetPriority=High  VelocityTargetValue=0  VelocityTargetValueUnits=deg/s
  link5_gripper_joint : sm_lib/Joints/Revolute Joint  JointMode=Normal  SenseConstraintForce=off  SenseConstraintForceX=off  SenseConstraintForceY=off  SenseConstraintForceZ=off  SenseConstraintTorque=off  SenseConstraintTorqueX=off  SenseConstraintTorqueY=off  SenseConstraintTorqueZ=off  SenseTotalForce=off  SenseTotalForceX=off  SenseTotalForceY=off  SenseTotalForceZ=off  SenseTotalTorque=off  SenseTotalTorqueX=off  SenseTotalTorqueY=off  SenseTotalTorqueZ=off  CompositeWrenchDir=FollowerOnBase  CompositeWrenchFrame=BaseFrame  EquilibriumPosition=0  EquilibriumPositionUnits=deg  SpringStiffness=0  SpringStiffnessUnits=N*m/deg  DampingCoefficient=fv6  DampingCoefficientUnits=N*m/(rad/s)  TorqueActuationMode=InputTorque  MotionActuationMode=ComputedMotion  SensePosition=on  SenseVelocity=on  SenseAcceleration=on  SenseTorqueForce=off  SenseLowerLimitTorqueForce=off  SenseUpperLimitTorqueForce=off  LowerLimitSpecify=on  LowerLimitBound=J6_lower_limit  LowerLimitBoundUnits=deg  LowerLimitStiffness=1e4  LowerLimitStiffnessUnits=N*m/deg  LowerLimitDamping=10  LowerLimitDampingUnits=N*m/(deg/s)  LowerLimitTransitionRegionWidth=0.1  LowerLimitTransitionRegionWidthUnits=deg  UpperLimitSpecify=on  UpperLimitBound=J6_upper_limit  UpperLimitBoundUnits=deg  UpperLimitStiffness=1e4  UpperLimitStiffnessUnits=N*m/deg  UpperLimitDamping=10  UpperLimitDampingUnits=N*m/(deg/s)  UpperLimitTransitionRegionWidth=0.1  UpperLimitTransitionRegionWidthUnits=deg  PositionTargetSpecify=on  PositionTargetPriority=High  PositionTargetValue=th6_0  PositionTargetValueUnits=deg  VelocityTargetSpecify=off  VelocityTargetPriority=High  VelocityTargetValue=0  VelocityTargetValueUnits=deg/s
  ConnB : PMIOPort  Side=Left
  q : Outport
  dq : Outport  Port=2
  ddq : Outport  Port=3
  wires:
  PS-Simulink Converter23/1 -> [ddth2]
  PS-Simulink Converter19/1 -> [dth1]
  [tau1] -> Simulink-PS Converter6/1
  PS-Simulink Converter30/1 -> [th5]
  PS-Simulink Converter35/1 -> [ddth6]
  PS-Simulink Converter34/1 -> [dth6]
  PS-Simulink Converter31/1 -> [dth5]
  [tau6] -> Simulink-PS Converter11/1
  [ddth1] -> Mux2/1
  PS-Simulink Converter32/1 -> [ddth5]
  [tau2] -> Simulink-PS Converter7/1
  PS-Simulink Converter26/1 -> [ddth3]
  [ddth4] -> Mux2/4
  PS-Simulink Converter24/1 -> [th3]
  PS-Simulink Converter27/1 -> [th4]
  PS-Simulink Converter25/1 -> [dth3]
  [tau4] -> Simulink-PS Converter9/1
  PS-Simulink Converter18/1 -> [th1]
  [ddth2] -> Mux2/2
  u/1 -> Demux/1
  [ddth5] -> Mux2/5
  Demux/6 -> [tau6]
  [th6] -> Mux/6
  [th2] -> Mux/2
  Mux/1 -> q/1
  Mux1/1 -> dq/1
  [dth6] -> Mux1/6
  [dth2] -> Mux1/2
  Demux/3 -> [tau3]
  [dth5] -> Mux1/5
  [tau5] -> Simulink-PS Converter10/1
  [ddth6] -> Mux2/6
  PS-Simulink Converter33/1 -> [th6]
  PS-Simulink Converter22/1 -> [dth2]
  Demux/5 -> [tau5]
  [dth1] -> Mux1/1
  [dth3] -> Mux1/3
  [dth4] -> Mux1/4
  [th1] -> Mux/1
  PS-Simulink Converter21/1 -> [th2]
  PS-Simulink Converter28/1 -> [dth4]
  Mux2/1 -> ddq/1
  [th4] -> Mux/4
  [tau3] -> Simulink-PS Converter8/1
  PS-Simulink Converter29/1 -> [ddth4]
  Demux/1 -> [tau1]
  Demux/2 -> [tau2]
  Demux/4 -> [tau4]
  [th5] -> Mux/5
  PS-Simulink Converter20/1 -> [ddth1]
  [ddth3] -> Mux2/3
  [th3] -> Mux/3
  connections:
  base_erb145_joint/LConn1 -- ConnB/RConn1
  Simulink-PS Converter7/RConn1 -- erb145_link2_joint/LConn2
  erb145_link2_joint/RConn1 -- link2/LConn1
  Simulink-PS Converter6/RConn1 -- base_erb145_joint/LConn2
  erb145_link3/RConn1 -- erb145_link4_joint/LConn1
  erb115_link5/LConn1 -- link4_erb115_joint/RConn1
  Simulink-PS Converter8/RConn1 -- link2_erb145_joint/LConn2
  link4/RConn1 -- link4_erb115_joint/LConn1
  Simulink-PS Converter9/RConn1 -- erb145_link4_joint/LConn2
  base_erb145_joint/RConn3 -- PS-Simulink Converter19/LConn1
  link2/RConn1 -- link2_erb145_joint/LConn1
  PS-Simulink Converter18/LConn1 -- base_erb145_joint/RConn2
  erb115_link5/RConn1 -- link5_gripper_joint/LConn1
  Simulink-PS Converter11/RConn1 -- link5_gripper_joint/LConn2
  PS-Simulink Converter24/LConn1 -- link2_erb145_joint/RConn2
  erb145_link1/RConn1 -- erb145_link2_joint/LConn1
  erb145_link2_joint/RConn4 -- PS-Simulink Converter23/LConn1
  PS-Simulink Converter21/LConn1 -- erb145_link2_joint/RConn2
  PS-Simulink Converter33/LConn1 -- link5_gripper_joint/RConn2
  erb145_link4_joint/RConn1 -- link4/LConn1
  link4_erb115_joint/RConn3 -- PS-Simulink Converter31/LConn1
  PS-Simulink Converter34/LConn1 -- link5_gripper_joint/RConn3
  link2_erb145_joint/RConn3 -- PS-Simulink Converter25/LConn1
  PS-Simulink Converter30/LConn1 -- link4_erb115_joint/RConn2
  PS-Simulink Converter29/LConn1 -- erb145_link4_joint/RConn4
  link2_erb145_joint/RConn4 -- PS-Simulink Converter26/LConn1
  PS-Simulink Converter27/LConn1 -- erb145_link4_joint/RConn2
  gripper/LConn1 -- link5_gripper_joint/RConn1
  Simulink-PS Converter10/RConn1 -- link4_erb115_joint/LConn2
  link4_erb115_joint/RConn4 -- PS-Simulink Converter32/LConn1
  PS-Simulink Converter22/LConn1 -- erb145_link2_joint/RConn3
  base_erb145_joint/RConn1 -- erb145_link1/LConn1
  PS-Simulink Converter28/LConn1 -- erb145_link4_joint/RConn3
  PS-Simulink Converter35/LConn1 -- link5_gripper_joint/RConn4
  base_erb145_joint/RConn4 -- PS-Simulink Converter20/LConn1
  erb145_link3/LConn1 -- link2_erb145_joint/RConn1

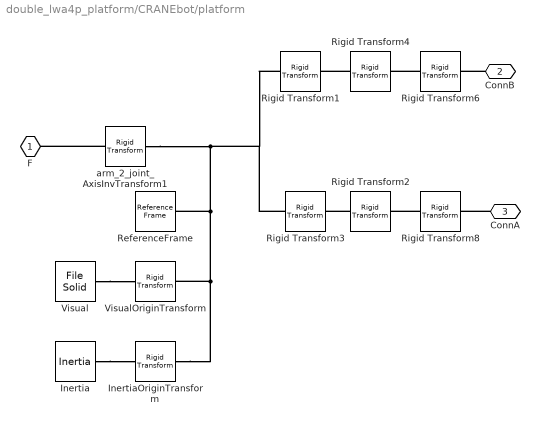
== system double_lwa4p_platform/CRANEbot/platform ==
  Inertia : sm_lib/Body Elements/Inertia  InertiaType=Custom  Mass=m_platform  MassUnits=kg  CenterOfMass=[0 0 0]  CenterOfMassUnits=m  MomentsOfInertia=[ixx_platform, iyy_platform, izz_platform]  MomentsOfInertiaUnits=kg*m^2  ProductsOfInertia=[iyz_platform, ixz_platform, ixy_platform]  ProductsOfInertiaUnits=kg*m^2  GraphicType=None  MarkerShape=Inertia  MarkerSize=20  GraphicVisPropType=SimpleVisualProperties  GraphicDiffuseColor=[0.5 0.5 0.5]  GraphicSpecularColor=[0.5 0.5 0.5 1.0]  GraphicAmbientColor=[0.15 0.15 0.15 1.0]  GraphicEmissiveColor=[0.0 0.0 0.0 1.0]  GraphicShininess=75  GraphicOpacity=1.0
  InertiaOriginTransform : sm_lib/Frames and Transforms/Rigid Transform  TranslationMethod=Cartesian  TranslationStandardOffset=0  TranslationLengthUnit=m  TranslationStandardAxis=+Z  TranslationCartesianOffset=inertial_disp_platform  TranslationROffset=0  TranslationROffsetUnits=m  TranslationZOffset=0  TranslationZOffsetUnits=m  TranslationThetaOffset=0  TranslationThetaOffsetUnits=deg  RotationMethod=RotationSequence  RotationAngleUnits=deg  RotationStandardAxis=+Z  RotationAngle=0.0  RotationArbitraryAxis=[0 0 1]  FollAlignAxisA=+X  BaseAlignAxisA=+Y  FollAlignAxisB=+Y  BaseAlignAxisB=+Z  RotationSequenceAxes=BaseAxes  RotationSequence=XYZ  RotationSequenceAngles=[0, 0, 0]  RotationSequenceAnglesUnits=rad  RotationMatrix=[1 0 0; 0 1 0; 0 0 1]
  ReferenceFrame : sm_lib/Frames and Transforms/Reference Frame
  Rigid Transform1 : sm_lib/Frames and Transforms/Rigid Transform  TranslationMethod=Cartesian  TranslationStandardOffset=4  TranslationLengthUnit=m  TranslationStandardAxis=-Y  TranslationCartesianOffset=[0 offB 0]  TranslationROffset=0  TranslationROffsetUnits=m  TranslationZOffset=0  TranslationZOffsetUnits=m  TranslationThetaOffset=0  TranslationThetaOffsetUnits=deg  RotationMethod=None  RotationAngleUnits=deg  RotationStandardAxis=+X  RotationAngle=180  RotationArbitraryAxis=[0 0 1]  FollAlignAxisA=+X  BaseAlignAxisA=+Y  FollAlignAxisB=+Y  BaseAlignAxisB=+Z  RotationSequenceAxes=FollowerAxes  RotationSequence=XYX  RotationSequenceAngles=[0 0 0]  RotationSequenceAnglesUnits=deg  RotationMatrix=[1 0 0; 0 1 0; 0 0 1]
  Rigid Transform2 : sm_lib/Frames and Transforms/Rigid Transform  TranslationMethod=Cartesian  TranslationStandardOffset=4  TranslationLengthUnit=m  TranslationStandardAxis=-Y  TranslationCartesianOffset=[0 0 0]  TranslationROffset=0  TranslationROffsetUnits=m  TranslationZOffset=0  TranslationZOffsetUnits=m  TranslationThetaOffset=0  TranslationThetaOffsetUnits=deg  RotationMethod=StandardAxis  RotationAngleUnits=deg  RotationStandardAxis=+Y  RotationAngle=180  RotationArbitraryAxis=[0 0 1]  FollAlignAxisA=+X  BaseAlignAxisA=+Y  FollAlignAxisB=+Y  BaseAlignAxisB=+Z  RotationSequenceAxes=FollowerAxes  RotationSequence=XYX  RotationSequenceAngles=[0 0 0]  RotationSequenceAnglesUnits=deg  RotationMatrix=[1 0 0; 0 1 0; 0 0 1]
  Rigid Transform3 : sm_lib/Frames and Transforms/Rigid Transform  TranslationMethod=Cartesian  TranslationStandardOffset=4  TranslationLengthUnit=m  TranslationStandardAxis=-Y  TranslationCartesianOffset=[0 offA 0]  TranslationROffset=0  TranslationROffsetUnits=m  TranslationZOffset=0  TranslationZOffsetUnits=m  TranslationThetaOffset=0  TranslationThetaOffsetUnits=deg  RotationMethod=None  RotationAngleUnits=deg  RotationStandardAxis=+X  RotationAngle=180  RotationArbitraryAxis=[0 0 1]  FollAlignAxisA=+X  BaseAlignAxisA=+Y  FollAlignAxisB=+Y  BaseAlignAxisB=+Z  RotationSequenceAxes=FollowerAxes  RotationSequence=XYX  RotationSequenceAngles=[0 0 0]  RotationSequenceAnglesUnits=deg  RotationMatrix=[1 0 0; 0 1 0; 0 0 1]
  Rigid Transform4 : sm_lib/Frames and Transforms/Rigid Transform  TranslationMethod=Cartesian  TranslationStandardOffset=4  TranslationLengthUnit=m  TranslationStandardAxis=-Y  TranslationCartesianOffset=[0 0 0]  TranslationROffset=0  TranslationROffsetUnits=m  TranslationZOffset=0  TranslationZOffsetUnits=m  TranslationThetaOffset=0  TranslationThetaOffsetUnits=deg  RotationMethod=StandardAxis  RotationAngleUnits=deg  RotationStandardAxis=+Y  RotationAngle=180  RotationArbitraryAxis=[0 0 1]  FollAlignAxisA=+X  BaseAlignAxisA=+Y  FollAlignAxisB=+Y  BaseAlignAxisB=+Z  RotationSequenceAxes=FollowerAxes  RotationSequence=XYX  RotationSequenceAngles=[0 0 0]  RotationSequenceAnglesUnits=deg  RotationMatrix=[1 0 0; 0 1 0; 0 0 1]
  Rigid Transform6 : sm_lib/Frames and Transforms/Rigid Transform  TranslationMethod=Cartesian  TranslationStandardOffset=4  TranslationLengthUnit=m  TranslationStandardAxis=-Y  TranslationCartesianOffset=[0 0 0.633]  TranslationROffset=0  TranslationROffsetUnits=m  TranslationZOffset=0  TranslationZOffsetUnits=m  TranslationThetaOffset=0  TranslationThetaOffsetUnits=deg  RotationMethod=StandardAxis  RotationAngleUnits=deg  RotationStandardAxis=+Z  RotationAngle=90  RotationArbitraryAxis=[0 0 1]  FollAlignAxisA=+X  BaseAlignAxisA=+Y  FollAlignAxisB=+Y  BaseAlignAxisB=+Z  RotationSequenceAxes=FollowerAxes  RotationSequence=XYX  RotationSequenceAngles=[0 0 0]  RotationSequenceAnglesUnits=deg  RotationMatrix=[1 0 0; 0 1 0; 0 0 1]
  Rigid Transform8 : sm_lib/Frames and Transforms/Rigid Transform  TranslationMethod=Cartesian  TranslationStandardOffset=4  TranslationLengthUnit=m  TranslationStandardAxis=-Y  TranslationCartesianOffset=[0 0 0.633]  TranslationROffset=0  TranslationROffsetUnits=m  TranslationZOffset=0  TranslationZOffsetUnits=m  TranslationThetaOffset=0  TranslationThetaOffsetUnits=deg  RotationMethod=StandardAxis  RotationAngleUnits=deg  RotationStandardAxis=+Z  RotationAngle=-90  RotationArbitraryAxis=[0 0 1]  FollAlignAxisA=+X  BaseAlignAxisA=+Y  FollAlignAxisB=+Y  BaseAlignAxisB=+Z  RotationSequenceAxes=FollowerAxes  RotationSequence=XYX  RotationSequenceAngles=[0 0 0]  RotationSequenceAnglesUnits=deg  RotationMatrix=[1 0 0; 0 1 0; 0 0 1]
  Visual : sm_lib/Body Elements/File Solid  ExtGeomFileName=platform_hook6_schunkbase.stl  UnitType=Custom  ExtGeomFileUnits=m  StepReaderType=HEX  ExportConvexHullGeometry=off  InertiaType=Custom  Mass=0  MassUnits=kg  CenterOfMass=[0, 0, 0]  CenterOfMassUnits=m  MomentsOfInertia=[0, 0, 0]  MomentsOfInertiaUnits=kg*m^2  ProductsOfInertia=[0, 0, 0]  ProductsOfInertiaUnits=kg*m^2  BasedOnType=DensityFromFile  Density=1000  DensityUnits=kg/m^3  DoExposeReferenceFrame=on  SerializedFrames=<Frames/>  GraphicType=FromGeometry  MarkerShape=Sphere  MarkerSize=10  GraphicVisPropType=SimpleVisualProperties  GraphicDiffuseColor=[0.6 0.6 0.6]  GraphicSpecularColor=[0.5 0.5 0.5 1.0]  GraphicAmbientColor=[0.15 0.15 0.15 1.0]  GraphicEmissiveColor=[0.0 0.0 0.0 1.0]  GraphicShininess=75  GraphicOpacity=1
  VisualOriginTransform : sm_lib/Frames and Transforms/Rigid Transform  TranslationMethod=Cartesian  TranslationStandardOffset=0  TranslationLengthUnit=m  TranslationStandardAxis=+Z  TranslationCartesianOffset=[0, 0, 0]  TranslationROffset=0  TranslationROffsetUnits=m  TranslationZOffset=0  TranslationZOffsetUnits=m  TranslationThetaOffset=0  TranslationThetaOffsetUnits=deg  RotationMethod=RotationSequence  RotationAngleUnits=deg  RotationStandardAxis=+Z  RotationAngle=0.0  RotationArbitraryAxis=[0 0 1]  FollAlignAxisA=+X  BaseAlignAxisA=+Y  FollAlignAxisB=+Y  BaseAlignAxisB=+Z  RotationSequenceAxes=BaseAxes  RotationSequence=XYZ  RotationSequenceAngles=[0, 0, 0]  RotationSequenceAnglesUnits=rad  RotationMatrix=[1 0 0; 0 1 0; 0 0 1]
  arm_2_joint_AxisInvTransform1 : sm_lib/Frames and Transforms/Rigid Transform  TranslationMethod=StandardAxis  TranslationStandardOffset=0.15111175  TranslationLengthUnit=m  TranslationStandardAxis=+Z  TranslationCartesianOffset=[0, 0, 0]  TranslationROffset=0  TranslationROffsetUnits=m  TranslationZOffset=0  TranslationZOffsetUnits=m  TranslationThetaOffset=0  TranslationThetaOffsetUnits=deg  RotationMethod=None  RotationAngleUnits=rad  RotationStandardAxis=+Z  RotationAngle=0  RotationArbitraryAxis=[1, 0, 0]  FollAlignAxisA=+X  BaseAlignAxisA=+Y  FollAlignAxisB=+Y  BaseAlignAxisB=+Z  RotationSequenceAxes=FollowerAxes  RotationSequence=XYX  RotationSequenceAngles=[0 0 0]  RotationSequenceAnglesUnits=deg  RotationMatrix=[1 0 0; 0 1 0; 0 0 1]
  F : PMIOPort  Side=Left
  ConnB : PMIOPort  Port=2  Side=Right
  ConnA : PMIOPort  Port=3  Side=Right
  connections:
  Inertia/RConn1 -- InertiaOriginTransform/RConn1
  Visual/RConn1 -- VisualOriginTransform/RConn1
  arm_2_joint_AxisInvTransform1/RConn1 -- F/RConn1
  InertiaOriginTransform/LConn1 -- VisualOriginTransform/LConn1 -- ReferenceFrame/RConn1 -- Rigid Transform3/LConn1 -- Rigid Transform1/LConn1 -- arm_2_joint_AxisInvTransform1/LConn1
  ConnA/RConn1 -- Rigid Transform8/RConn1
  ConnB/RConn1 -- Rigid Transform6/RConn1
  Rigid Transform8/LConn1 -- Rigid Transform2/RConn1
  Rigid Transform6/LConn1 -- Rigid Transform4/RConn1
  Rigid Transform2/LConn1 -- Rigid Transform3/RConn1
  Rigid Transform4/LConn1 -- Rigid Transform1/RConn1
